simulink model "file5"  (R2023a)
settings: Solver=VariableStepAuto  StartTime=0.0  StopTime=1.0  RelTol=1e-3
libraries: simulink_extras x7, spsFourierLib x6, spsDistributedParametersLineLib x2, spsSequenceAnalyzerLib x1, spsThreePhaseSeriesRLCLoadLib x1, spsThreePhaseVIMeasurementLib x1, spsThreePhaseFaultLib x1, spsThreePhaseSourceLib x1, sps_lib x1
settings Model: Creator=Dell  LastModifiedBy=Dell
settings DataIOCC: ReturnWorkspaceOutputs=off

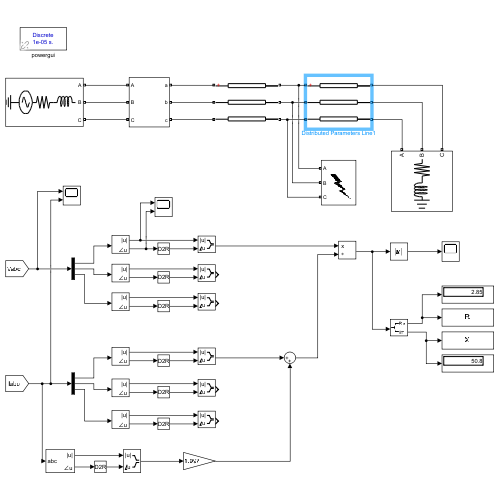
[thumbnail: Simulink's stored preview of the top-level diagram]
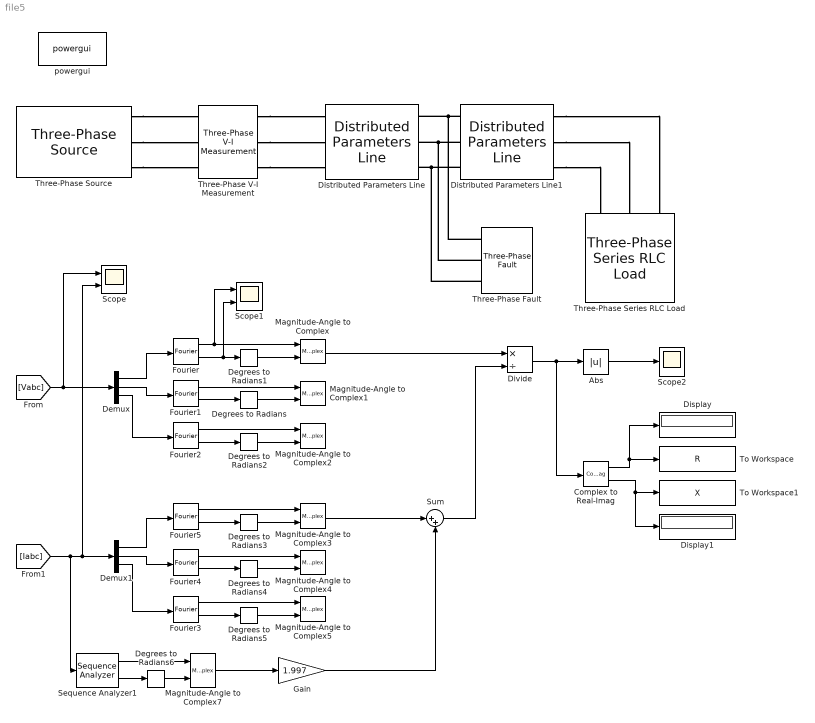
== system file5 ==
  Abs : Abs  SaturateOnIntegerOverflow=off
  Complex to Real-Imag : ComplexToRealImag
  Degrees to Radians{,1..6} (7 alike) : simulink_extras/Transformations/Degrees to Radians
  Demux : Demux  Outputs=3
  Demux1 : Demux  Outputs=3
  Display : Display
  Display1 : Display
  Distributed Parameters Line : spsDistributedParametersLineLib/Distributed Parameters Line  Phases=3  Length=180  Frequency=50  Resistance=[0.01537, 0.04612]  Inductance=[0.8858e-3, 2.6547e-3]  Capacitance=[13.06e-9, 4.3551e-9]  x1=[-0.00062 -1.5012663127771e-08 244533.444311894 -260368.233869218;-0.00061 -1.499271194952e-08 245350.207173951 -259598.725796012;-0.0006 -1.49726127992549e-08 246164.548528516 -258826.655588187;-0.00059 -1.49523658753461e-08 246976.460338367 -258052.030865763;-0.00058 -1.49319713776227e-08 247785.934590263 -257274.859273975;-0.00057 -1.491142950737e-08 248592.963295019 -256495.148483192;-0.00056 -1.48907404673281e-08 249397.538487589 -255712.906188844;-0.00055 -1.48699044616894e-08 250199.65222714 -254928.140111348;-0.00054 -1.48489216960969e-08 250999.296597134 -254140.857996027;-0.00053 -1.48277923776421e-08 251796.463705402 -253351.067613039;-0.00052 -1.48065167148626e-08 252591.145684228 -252558.776757296;-0.00051 -1.47850949177409e-08 253383.334690421 -251763.993248388;-0.0005 -1.47635271977012e-08 254173.022905396 -250966.724930508;-0.00049 -1.47418137676084e-08 254960.202535248 -250166.979672372;-0.00048 -1.47199548417653e-08 255744.865810833 -249364.765367144;-0.00047 -1.46979506359105e-08 256527.004987841 -248560.089932353;-0.00046 -1.46758013672167e-08 257306.612346874 -247752.961309823;-0.00045 -1.46535072542884e-08 258083.680193522 -246943.387465587;-0.00044 -1.46310685171592e-08 258858.200858439 -246131.376389812;-0.00043 -1.46084853772907e-08 259630.166697419 -245316.936096719;-0.00042 -1.45857580575691e-08 260399.57009147 -244500.074624505;-0.00041 -1.4562886782304e-08 261166.403446892 -243680.800035263;-0.0004 -1.45398717772257e-08 261930.659195349 -242859.120414903;-0.00039 -1.45167132694828e-08 262692.329793946 -242035.04387307;-0.00038 -1.44934114876407e-08 263451.407725301 -241208.578543068;-0.00037 -1.44699666616784e-08 264207.885497621 -240379.732581775;-0.00036 -1.44463790229869e-08 264961.755644776 -239548.514169568;-0.00035 -1.44226488043667e-08 265713.010726373 -238714.931510235;-0.00034 -1.43987762400254e-08 266461.643327826 -237878.992830901;-0.00033 -1.43747615655757e-08 267207.646060435 -237040.706381943;-0.00032 -1.43506050180327e-08 267951.011561453 -236200.080436911;-0.00031 -1.43263068358117e-08 268691.732494163 -235357.123292442;-0.0003 -1.43018672587259e-08 269429.801547949 -234511.843268185;-0.00029 -1.42772865279843e-08 270165.211438366 -233664.24870671;-0.00028 -1.42525648861886e-08 270897.954907217 -232814.347973435;-0.00027 -1.42277025773314e-08 271628.024722619 -231962.149456536;-0.00026 -1.42026998467938e-08 272355.413679077 -231107.661566869;-0.00025 -1.41775569413426e-08 273080.114597557 -230250.892737884;-0.00024 -1.4152274109128e-08 273802.120325553 -229391.851425544;-0.00023 -1.41268515996815e-08 274521.423737159 -228530.54610824;-0.00022 -1.4101289663913e-08 275238.017733142 -227666.985286707;-0.00021 -1.40755885541083e-08 275951.895241008 -226801.177483942;-0.0002 -1.40497485239272e-08 276663.049215074 -225933.131245119;-0.00019 -1.40237698284003e-08 277371.472636538 -225062.855137503;-0.00018 -1.39976527239268e-08 278077.158513547 -224190.357750369;-0.00017 -1.3971397468272e-08 278780.099881265 -223315.647694913;-0.00016 -1.39450043205647e-08 279480.289801945 -222438.73360417;-0.00015 -1.39184735412945e-08 280177.721364996 -221559.624132929;-0.00014 -1.38918053923097e-08 280872.387687049 -220678.327957645;-0.00013 -1.38650001368139e-08 281564.281912028 -219794.853776355;-0.00012 -1.38380580393643e-08 282253.397211218 -218909.210308593;-0.00011 -1.38109793658685e-08 282939.726783327 -218021.406295303;-0.0001 -1.37837643835821e-08 283623.26385456 -217131.450498752;-9e-05 -1.3756413361106e-08 284304.001678682 -216239.351702443;-8e-05 -1.37289265683836e-08 284981.933537085 -215345.118711033;-7e-05 -1.37013042766987e-08 285657.052738857 -214448.760350239;-6e-05 -1.36735467586719e-08 286329.352620842 -213550.285466757;-5e-05 -1.36456542882589e-08 286998.826547713 -212649.702928172;-4e-05 -1.36176271407471e-08 287665.467912032 -211747.021622868;-3e-05 -1.3589465592753e-08 288329.270134318 -210842.250459947;-2e-05 -1.35611699222198e-08 288990.226663111 -209935.398369134;-1e-05 -1.35327404084143e-08 289648.330975037 -209026.474300694]  x2=[-0.00062 -3.49971587945636e-08 233917.881307607 -271109.465273069;-0.00061 -3.49465554699949e-08 234768.441073486 -270373.253913944;-0.0006 -3.48956072370321e-08 235616.683769632 -269634.374079957;-0.00059 -3.48443145985138e-08 236462.601024231 -268892.833063553;-0.00058 -3.47926780606777e-08 237306.184488421 -268148.638183444;-0.00057 -3.47406981331555e-08 238147.425836375 -267401.796784531;-0.00056 -3.46883753289681e-08 238986.31676538 -266652.316237839;-0.00055 -3.46357101645204e-08 239822.848995922 -265900.203940438;-0.00054 -3.45827031595965e-08 240657.014271764 -265145.467315372;-0.00053 -3.45293548373539e-08 241488.804360033 -264388.113811587;-0.00052 -3.44756657243192e-08 242318.211051295 -263628.150903857;-0.00051 -3.44216363503822e-08 243145.226159642 -262865.586092708;-0.0005 -3.43672672487909e-08 243969.841522769 -262100.426904347;-0.00049 -3.43125589561466e-08 244792.049002054 -261332.680890588;-0.00048 -3.42575120123979e-08 245611.840482643 -260562.355628772;-0.00047 -3.42021269608359e-08 246429.207873523 -259789.458721699;-0.00046 -3.41464043480888e-08 247244.143107609 -259013.99779755;-0.00045 -3.40903447241162e-08 248056.638141819 -258235.980509811;-0.00044 -3.40339486422041e-08 248866.684957155 -257455.414537198;-0.00043 -3.39772166589589e-08 249674.275558782 -256672.307583583;-0.00042 -3.39201493343024e-08 250479.401976108 -255886.667377915;-0.00041 -3.38627472314662e-08 251282.056262858 -255098.501674145;-0.0004 -3.38050109169857e-08 252082.230497159 -254307.818251151;-0.00039 -3.3746940960695e-08 252879.916781615 -253514.62491266;-0.00038 -3.36885379357213e-08 253675.107243385 -252718.929487168;-0.00037 -3.36298024184788e-08 254467.794034258 -251920.739827869;-0.00036 -3.35707349886633e-08 255257.969330738 -251120.063812573;-0.00035 -3.35113362292465e-08 256045.625334111 -250316.909343628;-0.00034 -3.34516067264702e-08 256830.754270533 -249511.284347845;-0.00033 -3.33915470698405e-08 257613.348391097 -248703.196776417;-0.00032 -3.3331157852122e-08 258393.399971914 -247892.654604843;-0.00031 -3.32704396693317e-08 259170.901314192 -247079.665832845;-0.0003 -3.32093931207337e-08 259945.844744305 -246264.238484297;-0.00029 -3.31480188088328e-08 260718.222613875 -245446.380607135;-0.00028 -3.30863173393687e-08 261488.027299844 -244626.100273287;-0.00027 -3.30242893213099e-08 262255.251204551 -243803.405578589;-0.00026 -3.2961935366848e-08 263019.886755805 -242978.304642706;-0.00025 -3.28992560913912e-08 263781.926406962 -242150.80560905;-0.00024 -3.28362521135588e-08 264541.362636998 -241320.916644703;-0.00023 -3.27729240551746e-08 265298.187950585 -240488.645940334;-0.00022 -3.27092725412609e-08 266052.394878162 -239654.001710118;-0.00021 -3.26452982000325e-08 266803.975976011 -238816.992191658;-0.0002 -3.25810016628903e-08 267552.923826331 -237977.6256459;-0.00019 -3.25163835644151e-08 268299.231037308 -237135.910357051;-0.00018 -3.24514445423616e-08 269042.890243191 -236291.854632503;-0.00017 -3.23861852376517e-08 269783.894104365 -235445.466802745;-0.00016 -3.23206062943682e-08 270522.235307419 -234596.755221283;-0.00015 -3.2254708359749e-08 271257.906565226 -233745.728264557;-0.00014 -3.218849208418e-08 271990.900617006 -232892.39433186;-0.00013 -3.21219581211892e-08 272721.210228405 -232036.761845253;-0.00012 -3.20551071274399e-08 273448.82819156 -231178.839249484;-0.00011 -3.19879397627244e-08 274173.747325177 -230318.635011903;-0.0001 -3.19204566899575e-08 274895.960474596 -229456.157622377;-9e-05 -3.18526585751699e-08 275615.460511865 -228591.415593211;-8e-05 -3.17845460875016e-08 276332.240335809 -227724.417459058;-7e-05 -3.17161198991954e-08 277046.292872102 -226855.171776842;-6e-05 -3.164738068559e-08 277757.611073331 -225983.687125665;-5e-05 -3.15783291251139e-08 278466.187919075 -225109.97210673;-4e-05 -3.1508965899278e-08 279172.016415965 -224234.035343251;-3e-05 -3.14392916926693e-08 279875.08959776 -223355.885480369;-2e-05 -3.13693071929442e-08 280575.40052541 -222475.531185071;-1e-05 -3.12990130908214e-08 281272.94228713 -221592.981146096]  x3=[-0.00062 -9.21383868334256e-11 609.984975645492 -882.14982281352;-0.00061 -9.2525462962632e-11 612.753316336787 -880.229148416152;-0.0006 -9.2911625902873e-11 615.515609400229 -878.299786512453;-0.00059 -9.32968718428763e-11 618.271827573099 -876.361756144445;-0.00058 -9.368119698042e-11 621.021943652638 -874.415076439705;-0.00057 -9.40645975223701e-11 623.76593049631 -872.459766611176;-0.00056 -9.4447069684718e-11 626.503761022072 -870.495845956978;-0.00055 -9.4828609692618e-11 629.235408208643 -868.523333860213;-0.00054 -9.52092137804242e-11 631.960845095767 -866.54224978878;-0.00053 -9.55888781917279e-11 634.680044784483 -864.552613295178;-0.00052 -9.59675991793946e-11 637.392980437388 -862.554444016318;-0.00051 -9.63453730056011e-11 640.099625278902 -860.547761673322;-0.0005 -9.67221959418723e-11 642.799952595533 -858.532586071336;-0.00049 -9.70980642691178e-11 645.493935736141 -856.508937099329;-0.00048 -9.74729742776691e-11 648.181548112199 -854.476834729899;-0.00047 -9.78469222673157e-11 650.862763198059 -852.436299019077;-0.00046 -9.82199045473419e-11 653.53755453121 -850.387350106126;-0.00045 -9.85919174365632e-11 656.205895712542 -848.330008213345;-0.00044 -9.89629572633626e-11 658.867760406604 -846.264293645867;-0.00043 -9.93330203657267e-11 661.523122341867 -844.190226791462;-0.00042 -9.97021030912822e-11 664.171955310979 -842.107828120332;-0.00041 -1.00070201797332e-10 666.81423317103 -840.017118184911;-0.0004 -1.00437312850889e-10 669.449929843804 -837.918117619662;-0.00039 -1.00803432628717e-10 672.079019316037 -835.810847140873;-0.00038 -1.01168557517361e-10 674.701475639679 -833.695327546454;-0.00037 -1.01532683913186e-10 677.317272932145 -831.571579715728;-0.00036 -1.0189580822241e-10 679.926385376571 -829.439624609229;-0.00035 -1.02257926861145e-10 682.528787222071 -827.299483268494;-0.00034 -1.02619036255425e-10 685.124452783988 -825.151176815853;-0.00033 -1.02979132841245e-10 687.713356444153 -822.994726454224;-0.00032 -1.033382130646e-10 690.295472651131 -820.830153466902;-0.00031 -1.0369627338151e-10 692.870775920477 -818.657479217347;-0.0003 -1.04053310258066e-10 695.439240834988 -816.476725148978;-0.00029 -1.04409320170458e-10 698.000842044952 -814.287912784956;-0.00028 -1.04764299605011e-10 700.5555542684 -812.091063727977;-0.00027 -1.05118245058223e-10 703.103352291353 -809.886199660053;-0.00026 -1.05471153036793e-10 705.644210968072 -807.673342342302;-0.00025 -1.05823020057664e-10 708.17810522131 -805.452513614734;-0.00024 -1.06173842648049e-10 710.705010042553 -803.223735396031;-0.00023 -1.06523617345471e-10 713.224900492269 -800.987029683334;-0.00022 -1.06872340697796e-10 715.737751700158 -798.742418552025;-0.00021 -1.07220009263264e-10 718.243538865393 -796.48992415551;-0.0002 -1.07566619610526e-10 720.742237256865 -794.229568725001;-0.00019 -1.0791216831868e-10 723.233822213432 -791.961374569291;-0.00018 -1.08256651977298e-10 725.718269144155 -789.685364074542;-0.00017 -1.08600067186467e-10 728.195553528545 -787.401559704059;-0.00016 -1.08942410556816e-10 730.665650916807 -785.109983998068;-0.00015 -1.09283678709554e-10 733.128536930075 -782.810659573497;-0.00014 -1.09623868276503e-10 735.58418726066 -780.503609123749;-0.00013 -1.09962975900129e-10 738.032577672285 -778.188855418481;-0.00012 -1.10300998233577e-10 740.473684000323 -775.866421303378;-0.00011 -1.10637931940703e-10 742.907482152042 -773.536329699927;-0.0001 -1.10973773696107e-10 745.333948106835 -771.19860360519;-9e-05 -1.11308520185166e-10 747.753057916465 -768.853266091582;-8e-05 -1.11642168104068e-10 750.164787705292 -766.500340306635;-7e-05 -1.11974714159843e-10 752.569113670519 -764.139849472779;-6e-05 -1.12306155070395e-10 754.966012082419 -761.771816887104;-5e-05 -1.12636487564536e-10 757.355459284571 -759.396265921136;-4e-05 -1.12965708382018e-10 759.737431694097 -757.013220020605;-3e-05 -1.13293814273565e-10 762.111905801891 -754.62270270521;-2e-05 -1.13620802000903e-10 764.478858172851 -752.224737568393;-1e-05 -1.13946668336796e-10 766.838265446114 -749.819348277102]  x4=[-0.00062 2.45339486768157e-11 1016.71493304622 -1318.63984751096;-0.00061 2.49929807738273e-11 1020.85253820658 -1315.43924137912;-0.0006 2.54517662002087e-11 1024.98006796452 -1312.22565239304;-0.00059 2.59103004279329e-11 1029.097481583 -1308.99911226953;-0.00058 2.63685789314524e-11 1033.20473842479 -1305.75965285325;-0.00057 2.68265971877433e-11 1037.30179795294 -1302.50730611635;-0.00056 2.72843506763502e-11 1041.38861973111 -1299.24210415819;-0.00055 2.77418348794311e-11 1045.46516342404 -1295.96407920498;-0.00054 2.81990452818015e-11 1049.53138879787 -1292.67326360951;-0.00053 2.86559773709795e-11 1053.58725572061 -1289.3696898508;-0.00052 2.91126266372297e-11 1057.63272416249 -1286.0533905338;-0.00051 2.95689885736082e-11 1061.66775419636 -1282.72439838903;-0.0005 3.0025058676007e-11 1065.69230599811 -1279.3827462723;-0.00049 3.04808324431983e-11 1069.70633984704 -1276.02846716438;-0.00048 3.09363053768789e-11 1073.70981612625 -1272.66159417064;-0.00047 3.1391472981715e-11 1077.70269532305 -1269.28216052076;-0.00046 3.1846330765386e-11 1081.68493802933 -1265.89019956838;-0.00045 3.23008742386292e-11 1085.65650494197 -1262.4857447908;-0.00044 3.27550989152841e-11 1089.61735686321 -1259.0688297886;-0.00043 3.32090003123364e-11 1093.56745470102 -1255.63948828535;-0.00042 3.36625739499627e-11 1097.50675946955 -1252.19775412728;-0.00041 3.41158153515743e-11 1101.43523228945 -1248.74366128291;-0.0004 3.45687200438614e-11 1105.35283438827 -1245.27724384275;-0.00039 3.50212835568376e-11 1109.25952710086 -1241.79853601892;-0.00038 3.54735014238838e-11 1113.15527186975 -1238.30757214487;-0.00037 3.59253691817922e-11 1117.0400302455 -1234.80438667502;-0.00036 3.63768823708104e-11 1120.91376388713 -1231.28901418438;-0.00035 3.68280365346856e-11 1124.77643456243 -1227.76148936826;-0.00034 3.72788272207082e-11 1128.62800414841 -1224.22184704191;-0.00033 3.77292499797563e-11 1132.46843463164 -1220.67012214016;-0.00032 3.81793003663389e-11 1136.29768810862 -1217.10634971712;-0.00031 3.86289739386406e-11 1140.11572678616 -1213.53056494577;-0.0003 3.90782662585646e-11 1143.92251298175 -1209.94280311766;-0.00029 3.95271728917772e-11 1147.71800912396 -1206.34309964256;-0.00028 3.99756894077511e-11 1151.50217775278 -1202.73149004809;-0.00027 4.04238113798094e-11 1155.27498151998 -1199.10800997937;-0.00026 4.08715343851691e-11 1159.03638318952 -1195.4726951987;-0.00025 4.1318854004985e-11 1162.78634563788 -1191.82558158515;-0.00024 4.17657658243929e-11 1166.52483185444 -1188.16670513428;-0.00023 4.22122654325537e-11 1170.25180494185 -1184.49610195771;-0.00022 4.26583484226964e-11 1173.9672281164 -1180.81380828281;-0.00021 4.3104010392162e-11 1177.67106470836 -1177.11986045234;-0.0002 4.35492469424469e-11 1181.36327816236 -1173.41429492406;-0.00019 4.3994053679246e-11 1185.04383203774 -1169.69714827043;-0.00018 4.44384262124964e-11 1188.71269000891 -1165.96845717816;-0.00017 4.48823601564206e-11 1192.36981586574 -1162.22825844794;-0.00016 4.53258511295698e-11 1196.01517351386 -1158.47658899403;-0.00015 4.57688947548672e-11 1199.64872697508 -1154.71348584387;-0.00014 4.62114866596509e-11 1203.27044038767 -1150.93898613779;-0.00013 4.66536224757177e-11 1206.8802780068 -1147.15312712857;-0.00012 4.70952978393654e-11 1210.47820420482 -1143.3559461811;-0.00011 4.75365083914367e-11 1214.06418347166 -1139.54748077204;-0.0001 4.79772497773613e-11 1217.63818041514 -1135.7277684894;-9e-05 4.84175176471999e-11 1221.20015976136 -1131.89684703219;-8e-05 4.88573076556862e-11 1224.75008635503 -1128.05475421007;-7e-05 4.92966154622705e-11 1228.28792515979 -1124.20152794294;-6e-05 4.97354367311619e-11 1231.81364125861 -1120.33720626059;-5e-05 5.01737671313719e-11 1235.3271998541 -1116.46182730231;-4e-05 5.06116023367563e-11 1238.82856626884 -1112.57542931653;-3e-05 5.10489380260583e-11 1242.31770594577 -1108.67805066043;-2e-05 5.14857698829513e-11 1245.79458444849 -1104.76972979955;-1e-05 5.19220935960811e-11 1249.25916746161 -1100.85050530746]  x5=0.000612226228774952  V1=ones(3,3)  V2=ones(3,3)  I1=ones(3,3)  I2=ones(3,3)  nHarmo=1  Measurements=None  Decoupling=off  VsMag0=0  VrMag0=0  VsAngle0=0  VrAngle0=0  IsMag0=0  IrMag0=0  IsAngle0=0  IrAngle0=0
      settings: LibrarySourceBlock=sps_lib/Power Grid Elements/Distributed Parameters Line
  Distributed Parameters Line1 : spsDistributedParametersLineLib/Distributed Parameters Line  Phases=3  Length=20  Frequency=50  Resistance=[0.01537, 0.04612]  Inductance=[0.8858e-3, 2.6547e-3]  Capacitance=[13.06e-9, 4.3551e-9]  x1=[-7e-05 -3.17161198991954e-08 277046.292872102 -226855.171776842;-6e-05 -3.164738068559e-08 277757.611073331 -225983.687125665;-5e-05 -3.15783291251139e-08 278466.187919075 -225109.97210673;-4e-05 -3.1508965899278e-08 279172.016415965 -224234.035343251;-3e-05 -3.14392916926693e-08 279875.08959776 -223355.885480369;-2e-05 -3.13693071929442e-08 280575.40052541 -222475.531185071;-1e-05 -3.12990130908214e-08 281272.94228713 -221592.981146096]  x2=[-7e-05 -3.18206675334516e-08 275478.904456889 -227685.60642335;-6e-05 -3.17536269333259e-08 276192.839275957 -226819.041761977;-5e-05 -3.16862729377219e-08 276904.048183205 -225950.238488232;-4e-05 -3.16186062113963e-08 277612.524159289 -225079.205176853;-3e-05 -3.15506274221923e-08 278318.260211835 -224205.950424587;-2e-05 -3.14823372410332e-08 279021.249375515 -223330.482850106;-1e-05 -3.14137363419154e-08 279721.48471211 -222452.811093921]  x3=[-7e-05 -5.79979436811282e-12 889.372035170406 -609.251834918751;-6e-05 -5.73429399593093e-12 891.281664239268 -606.454788327944;-5e-05 -5.66873702858234e-12 893.18249671793 -603.651756273213;-4e-05 -5.60312411308783e-12 895.074513845941 -600.842766419352;-3e-05 -5.53745589702041e-12 896.957696949856 -598.027846489956;-2e-05 -5.47173302849883e-12 898.83202744342 -595.207024267148;-1e-05 -5.4059561561813e-12 900.697486827745 -592.380327591306]  x4=[-7e-05 -6.61450085738178e-11 1211.67408139744 -1157.18713339578;-6e-05 -6.60307178568883e-11 1215.30350664753 -1153.37484277978;-5e-05 -6.59157754434312e-11 1218.92093734265 -1149.55116881972;-4e-05 -6.58001824678818e-11 1222.52633778021 -1145.71614925372;-3e-05 -6.56839400710961e-11 1226.11967237638 -1141.86982193186;-2e-05 -6.55670494003395e-11 1229.70090566638 -1138.01222481586;-1e-05 -6.54495116092758e-11 1233.27000230489 -1134.14339597863]  x5=6.80251365305502e-05  V1=ones(3,3)  V2=ones(3,3)  I1=ones(3,3)  I2=ones(3,3)  nHarmo=1  Measurements=None  Decoupling=off  VsMag0=0  VrMag0=0  VsAngle0=0  VrAngle0=0  IsMag0=0  IrMag0=0  IsAngle0=0  IrAngle0=0
      settings: LibrarySourceBlock=sps_lib/Power Grid Elements/Distributed Parameters Line
  Divide : Product  Inputs=*/
  Fourier{,1..5} (6 alike) : spsFourierLib/Fourier  Freq=50  n=1  InInit=[0, 0]  Ts=0
  Gain : Gain  Gain=1.997
  Magnitude-Angle to Complex{,1..5,7} (7 alike) : MagnitudeAngleToComplex
  Scope : Scope  NumInputPorts=2
  Scope1 : Scope  NumInputPorts=2
  Scope2 : Scope
  Sequence Analyzer1 : spsSequenceAnalyzerLib/Sequence Analyzer  Freq=50  n=1  seq=Zero  InInit=[1, 0]  Ts=0
      settings: LibrarySourceBlock=sps_lib/Sensors and Measurements/Sequence Analyzer
  Sum : Sum  Inputs=|++
  Three-Phase Series RLC Load : spsThreePhaseSeriesRLCLoadLib/Three-Phase Series RLC Load  LConnTagsString=A|B|C  Configuration=Y (grounded)  NominalVoltage=345e3  Vabc=[1e3 1e3 1e3]  Vabcp=[1e3 1e3 1e3]  NominalFrequency=50  UnbalancedPower=off  ActivePower=100e6  InductivePower=40e6  CapacitivePower=0  Pabc=[10e3 9e3 11e3]  QLabc=[100 90 110]  QCabc=[100 90 110]  Pabcp=[10e3 9e3 11e3]  QLabcp=[100 90 110]  QCabcp=[100 90 110]  Measurements=None  LoadType=constant Z
  Three-Phase V-I Measurement : spsThreePhaseVIMeasurementLib/Three-Phase V-I Measurement  VoltageMeasurement=phase-to-ground  SetLabelV=on  LabelV=Vabc  Vpu=off  VpuLL=off  CurrentMeasurement=yes  SetLabelI=on  LabelI=Iabc  Ipu=off  Pbase=100e6  Vbase=500e3  OutputType=Complex  PhasorSimulation=off  PSBequivalent=0
  Three-Phase Fault : spsThreePhaseFaultLib/Three-Phase Fault  InitialStates=0  FaultA=on  FaultB=on  FaultC=on  GroundFault=off  SwitchTimes=0.7  External=off  SwitchStatus=NaN  FaultResistance=0.1  GroundResistance=0.01  SnubberResistance=1e6  SnubberCapacitance=inf  Measurements=None
  Three-Phase Source : spsThreePhaseSourceLib/Three-Phase Source  InternalConnection=Yg  VoltagePhases=off  Voltage=345e3  PhaseAngle=30  Voltage_phases=[25e3 25e3 25e3]/sqrt(3)  PhaseAngles_phases=[0 -120 +120]  Frequency=50  NonIdealSource=on  SpecifyImpedance=on  Resistance=0.8929  Inductance=16.58e-3  ShortCircuitLevel=1500e6  BaseVoltage=400e3  XRratio=10  BusType=swing  Pref=10e3  Qref=0  Prefabc=[10e3, 10e3, 10e3]  Qrefabc=[0, 0, 0]  Qmin=-inf  Qmax=inf
  To Workspace : ToWorkspace  VariableName=R  SampleTime=1e-4
      settings: Save2DSignal=2-D array (concatenate along first dimension)
  To Workspace1 : ToWorkspace  VariableName=X  SampleTime=1e-4
      settings: Save2DSignal=2-D array (concatenate along first dimension)
  powergui : sps_lib/powergui  Priority=1  SimulationMode=Discrete  SampleTime=1e-05  frequency=60  Iterations=50  frequencyindice=50  Pbase=100e6  ErrMax=1e-4  UnitsV=kV  UnitsW=MW  buscounter=0  FunctionMessages=off  echomessages=off  EnableUseOfTLC=off  CurrentSourceSwitches=off  DisableSnubberDevices=off  DisableRonSwitches=off  DisableVfSwitches=off  DisplayEquations=off  AutomaticDiscreteSolvers=off  SolverType=Tustin/Backward Euler (TBE)  Interpol=off  ExternalGateDelay=off  methode=off  Ts=100  x0status=blocks  SPID=on  SwTol=0  HookPort=off  NonlinearTolerance=1e-4  nMaxIteration=100  ContinueOnMaxIteration=off  RestoreLinks=warning  ResistiveCurrentMeasurement=off  Frange=[0:2:500]  Ylog=off  Xlog=on  ShowGrid=off  save=off  variable=ZData  structure=0  ZoomFFT=off  StartTime=0.0  cycles=1  DisplayStyle=1  fundamental=60  FreqAxis=off  MaxFrequency=1000  frequencyindicesteady=1  RmsSteady=1  display=off
  wires:
  [Iabc] -> Sequence Analyzer1/1, Demux1/1, Scope/2
  [Vabc] -> Scope/1, Demux/1
  Demux/1 -> Fourier/1
  Demux/2 -> Fourier1/1
  Demux/3 -> Fourier2/1
  Demux1/1 -> Fourier5/1
  Demux1/2 -> Fourier4/1
  Demux1/3 -> Fourier3/1
  Fourier1/2 -> Degrees to Radians/1
  Fourier/2 -> Scope1/2, Degrees to Radians1/1
  Fourier2/2 -> Degrees to Radians2/1
  Fourier5/2 -> Degrees to Radians3/1
  Fourier4/2 -> Degrees to Radians4/1
  Fourier3/2 -> Degrees to Radians5/1
  Fourier/1 -> Scope1/1, Magnitude-Angle to Complex/1
  Degrees to Radians1/1 -> Magnitude-Angle to Complex/2
  Fourier1/1 -> Magnitude-Angle to Complex1/1
  Degrees to Radians/1 -> Magnitude-Angle to Complex1/2
  Fourier2/1 -> Magnitude-Angle to Complex2/1
  Degrees to Radians2/1 -> Magnitude-Angle to Complex2/2
  Degrees to Radians3/1 -> Magnitude-Angle to Complex3/2
  Fourier5/1 -> Magnitude-Angle to Complex3/1
  Degrees to Radians4/1 -> Magnitude-Angle to Complex4/2
  Fourier4/1 -> Magnitude-Angle to Complex4/1
  Degrees to Radians5/1 -> Magnitude-Angle to Complex5/2
  Fourier3/1 -> Magnitude-Angle to Complex5/1
  Magnitude-Angle to Complex/1 -> Divide/1
  Magnitude-Angle to Complex3/1 -> Sum/1
  Sum/1 -> Divide/2
  Sequence Analyzer1/2 -> Degrees to Radians6/1
  Degrees to Radians6/1 -> Magnitude-Angle to Complex7/2
  Sequence Analyzer1/1 -> Magnitude-Angle to Complex7/1
  Magnitude-Angle to Complex7/1 -> Gain/1
  Gain/1 -> Sum/2
  Divide/1 -> Complex to Real-Imag/1, Abs/1
  Abs/1 -> Scope2/1
  Complex to Real-Imag/1 -> Display/1, To Workspace/1
  Complex to Real-Imag/2 -> Display1/1, To Workspace1/1
  connections:
  Three-Phase Source/RConn1 -- Three-Phase V-I Measurement/LConn1
  Three-Phase Source/RConn2 -- Three-Phase V-I Measurement/LConn2
  Three-Phase Source/RConn3 -- Three-Phase V-I Measurement/LConn3
  Distributed Parameters Line1/LConn1 -- Three-Phase Fault/LConn1 -- Distributed Parameters Line/RConn1
  Distributed Parameters Line1/LConn2 -- Three-Phase Fault/LConn2 -- Distributed Parameters Line/RConn2
  Distributed Parameters Line1/LConn3 -- Three-Phase Fault/LConn3 -- Distributed Parameters Line/RConn3
  Three-Phase V-I Measurement/RConn1 -- Distributed Parameters Line/LConn1
  Three-Phase V-I Measurement/RConn2 -- Distributed Parameters Line/LConn2
  Three-Phase V-I Measurement/RConn3 -- Distributed Parameters Line/LConn3
  Distributed Parameters Line1/RConn3 -- Three-Phase Series RLC Load/LConn1
  Distributed Parameters Line1/RConn2 -- Three-Phase Series RLC Load/LConn2
  Distributed Parameters Line1/RConn1 -- Three-Phase Series RLC Load/LConn3
